simulink model "problem_4_13"  (R2018b)
settings: Solver=VariableStepAuto  StartTime=0.0  StopTime=1000  RelTol=1e-3
values from neighbouring files (symbols this model uses):
  alpha = 0.001    [problem_4_13_params.m]
  beta = data.Data(:,5)    [problem_4_13_params.m]
  Gamma = diag([30, 5])    [problem_4_13_params.m]
  gamma = 0.01    [problem_4_13_params.m]
  k = data.Data(:,6)    [problem_4_13_params.m]
  lambda1 = -2    [problem_4_13_params.m]
  lambda2 = -2    [problem_4_13_params.m]
settings Model: Creator=cale  LastModifiedBy=cale

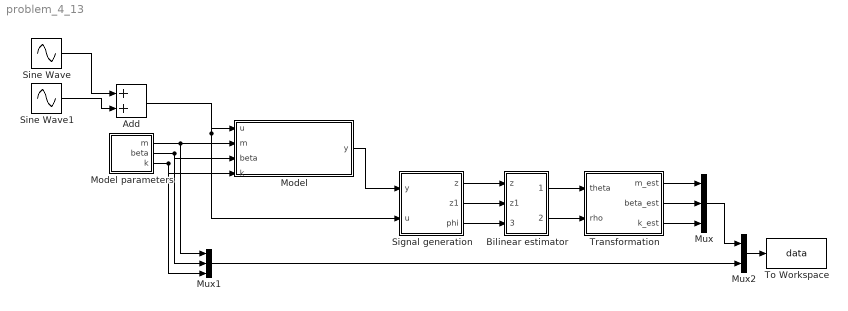
== system problem_4_13 ==
  Add : Sum
  Bilinear estimator : Subsystem
  Model : Subsystem
  Model parameters : Subsystem
  Mux : Mux  Inputs=3
  Mux1 : Mux  Inputs=3
  Mux2 : Mux  Inputs=2
  Signal generation : Subsystem
  Sine Wave : Sin  Frequency=0.1  SampleTime=0
  Sine Wave1 : Sin  Bias=20  Frequency=5  SampleTime=0
  To Workspace : ToWorkspace  VariableName=data  SaveFormat=Timeseries  SampleTime=-1
  Transformation : Subsystem
  wires:
  Model parameters/1(m) -> Mux1/1, Model/2(m)
  Model parameters/2(beta) -> Mux1/2, Model/3(beta)
  Model parameters/3(k) -> Mux1/3, Model/4(k)
  Model/1(y) -> Signal generation/1(y)
  Add/1 -> Signal generation/2(u), Model/1(u)
  Signal generation/1("z ") -> Bilinear estimator/1(z)
  Signal generation/2(z1) -> Bilinear estimator/2(z1)
  Signal generation/3(phi) -> Bilinear estimator/3(phi)
  Sine Wave/1 -> Add/1
  Sine Wave1/1 -> Add/2
  Bilinear estimator/1(theta) -> Transformation/1(theta)
  Bilinear estimator/2(rho) -> Transformation/2(rho)
  Transformation/1(m_est) -> Mux/1
  Transformation/2(beta_est) -> Mux/2
  Transformation/3(k_est) -> Mux/3
  Mux/1 -> Mux2/1
  Mux1/1 -> Mux2/2
  Mux2/1 -> To Workspace/1

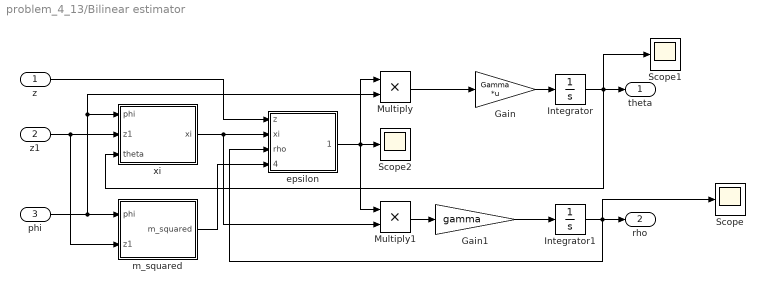
== system problem_4_13/Bilinear estimator ==
  z : Inport
  z1 : Inport  Port=2
  phi : Inport  Port=3
  Gain : Gain  Gain=Gamma  Multiplication=Matrix(K*u) (u vector)
  Gain1 : Gain  Gain=gamma
  Integrator : Integrator  InitialCondition=[10,1]
  Integrator1 : Integrator  InitialCondition=1
  Multiply : Product
  Multiply1 : Product
  Scope : Scope
  Scope1 : Scope
  Scope2 : Scope
  epsilon : Subsystem
  m_squared : Subsystem
  xi : Subsystem
  theta : Outport  PortDimensions=2
  rho : Outport  Port=2
  wires:
  Integrator/1 -> Scope1/1, xi/3(theta), theta/1
  phi/1 -> m_squared/1(phi), Multiply/2, xi/1(phi)
  z1/1 -> m_squared/2(z1), xi/2(z1)
  z/1 -> epsilon/1(z)
  xi/1(xi) -> epsilon/2(xi), Multiply1/2
  m_squared/1(m_squared) -> epsilon/4(m_squared)
  Multiply/1 -> Gain/1
  Gain/1 -> Integrator/1
  epsilon/1(epsilon) -> Scope2/1, Multiply/1, Multiply1/1
  Gain1/1 -> Integrator1/1
  Multiply1/1 -> Gain1/1
  Integrator1/1 -> Scope/1, epsilon/3(rho), rho/1

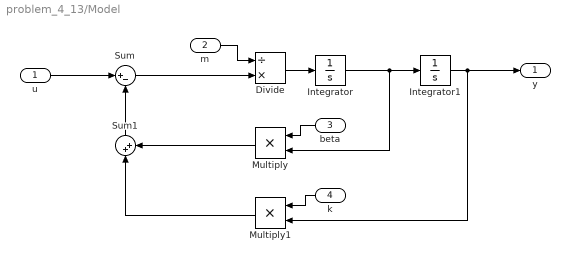
== system problem_4_13/Model ==
  u : Inport
  m : Inport  Port=2
  beta : Inport  Port=3
  k : Inport  Port=4
  Divide : Product  Inputs=/*
  Integrator : Integrator
  Integrator1 : Integrator
  Multiply : Product
  Multiply1 : Product
  Sum : Sum  Inputs=|+-
  Sum1 : Sum  Inputs=|++
  y : Outport
  wires:
  Integrator/1 -> Multiply/2, Integrator1/1
  Divide/1 -> Integrator/1
  m/1 -> Divide/1
  u/1 -> Sum/1
  Sum/1 -> Divide/2
  Sum1/1 -> Sum/2
  Multiply/1 -> Sum1/2
  beta/1 -> Multiply/1
  Integrator1/1 -> Multiply1/2, y/1
  k/1 -> Multiply1/1
  Multiply1/1 -> Sum1/1

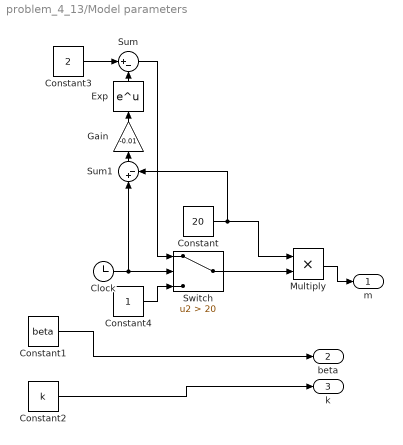
== system problem_4_13/Model parameters ==
  Clock : Clock
  Constant : Constant  Value=20
  Constant1 : Constant  Value=beta
  Constant2 : Constant  Value=k
  Constant3 : Constant  Value=2
  Constant4 : Constant
  Exp : Math  SaturateOnIntegerOverflow=on
  Gain : Gain  Gain=-0.01
  Multiply : Product
  Sum : Sum  Inputs=|+-
  Sum1 : Sum  Inputs=|+-
  Switch : Switch  Criteria=u2 > Threshold  Threshold=20
  m : Outport
  beta : Outport  Port=2
  k : Outport  Port=3
  wires:
  Constant1/1 -> beta/1
  Constant2/1 -> k/1
  Clock/1 -> Switch/2, Sum1/1
  Constant/1 -> Multiply/1, Sum1/2
  Multiply/1 -> m/1
  Constant3/1 -> Sum/1
  Exp/1 -> Sum/2
  Sum1/1 -> Gain/1
  Gain/1 -> Exp/1
  Sum/1 -> Switch/1
  Constant4/1 -> Switch/3
  Switch/1 -> Multiply/2

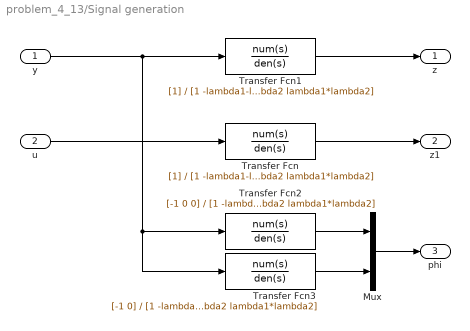
== system problem_4_13/Signal generation ==
  y : Inport
  u : Inport  Port=2
  Mux : Mux  Inputs=2
  Transfer Fcn : TransferFcn  Denominator=[1 -lambda1-lambda2 lambda1*lambda2]
  Transfer Fcn1 : TransferFcn  Denominator=[1 -lambda1-lambda2 lambda1*lambda2]
  Transfer Fcn2 : TransferFcn  Numerator=[-1 0 0]  Denominator=[1 -lambda1-lambda2 lambda1*lambda2]
  Transfer Fcn3 : TransferFcn  Numerator=[-1 0]  Denominator=[1 -lambda1-lambda2 lambda1*lambda2]
  "z " : Outport
  z1 : Outport  Port=2
  phi : Outport  Port=3  PortDimensions=2
  wires:
  Transfer Fcn/1 -> z1/1
  u/1 -> Transfer Fcn/1
  Transfer Fcn1/1 -> "z "/1
  Mux/1 -> phi/1
  Transfer Fcn2/1 -> Mux/1
  Transfer Fcn3/1 -> Mux/2
  y/1 -> Transfer Fcn3/1, Transfer Fcn2/1, Transfer Fcn1/1

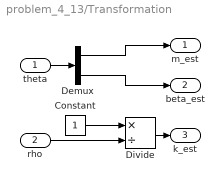
== system problem_4_13/Transformation ==
  theta : Inport
  rho : Inport  Port=2
  Constant : Constant
  Demux : Demux  Outputs=2
  Divide : Product  Inputs=*/
  m_est : Outport
  beta_est : Outport  Port=2
  k_est : Outport  Port=3
  wires:
  Demux/1 -> m_est/1
  theta/1 -> Demux/1
  Demux/2 -> beta_est/1
  rho/1 -> Divide/2
  Divide/1 -> k_est/1
  Constant/1 -> Divide/1

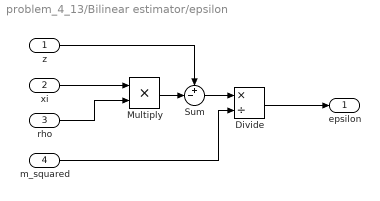
== system problem_4_13/Bilinear estimator/epsilon ==
  z : Inport
  xi : Inport  Port=2
  rho : Inport  Port=3
  m_squared : Inport  Port=4
  Divide : Product  Inputs=*/
  Multiply : Product
  Sum : Sum  Inputs=+-|
  epsilon : Outport
  wires:
  m_squared/1 -> Divide/2
  rho/1 -> Multiply/2
  Divide/1 -> epsilon/1
  Sum/1 -> Divide/1
  Multiply/1 -> Sum/2
  xi/1 -> Multiply/1
  z/1 -> Sum/1

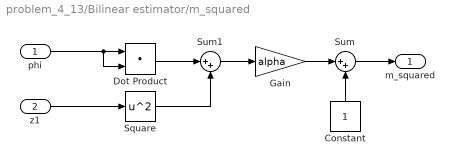
== system problem_4_13/Bilinear estimator/m_squared ==
  phi : Inport
  z1 : Inport  Port=2
  Constant : Constant
  Dot Product : DotProduct  InputSameDT=on  OutDataTypeStr=Inherit: Inherit via internal rule
  Gain : Gain  Gain=alpha
  Square : Math  Operator=square  SaturateOnIntegerOverflow=on
  Sum : Sum  Inputs=|++
  Sum1 : Sum  Inputs=|++
  m_squared : Outport
  wires:
  phi/1 -> Dot Product/2, Dot Product/1
  Sum/1 -> m_squared/1
  Constant/1 -> Sum/2
  Gain/1 -> Sum/1
  z1/1 -> Square/1
  Dot Product/1 -> Sum1/1
  Sum1/1 -> Gain/1
  Square/1 -> Sum1/2

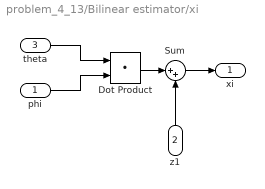
== system problem_4_13/Bilinear estimator/xi ==
  phi : Inport
  z1 : Inport  Port=2
  theta : Inport  Port=3
  Dot Product : DotProduct  InputSameDT=on  OutDataTypeStr=Inherit: Inherit via internal rule
  Sum : Sum  Inputs=|++
  xi : Outport
  wires:
  theta/1 -> Dot Product/1
  phi/1 -> Dot Product/2
  Dot Product/1 -> Sum/1
  Sum/1 -> xi/1
  z1/1 -> Sum/2
